simulink model "psb2rectifiers"  (Simulink 6.0)
settings: Solver=ode23tb  SolverMode=SingleTasking  StartTime=0.0  StopTime=0.1  RelTol=1e-3
InitFcn:
  | powericon('psbinitsys',bdroot);
libraries: powerlib2 x29
settings Model: Creator=sybille  LastModifiedBy=batserve  ExtModeTrigMode=oneshot  ExtModeArmWhenConnect=off  ExtModeAutoUpdateStatusClock=off
settings DataIOCC: LimitDataPoints=off  SignalLoggingName=sigsOut
settings OptimizationCC: BlockReduction=off  BooleanDataType=off
settings DebuggingCC: CheckExecutionContextPreStartOutputMsg=on  CheckExecutionContextRuntimeOutputMsg=on  SolverPrmCheckMsg=none
settings HardwareCC: TargetUnknown=on

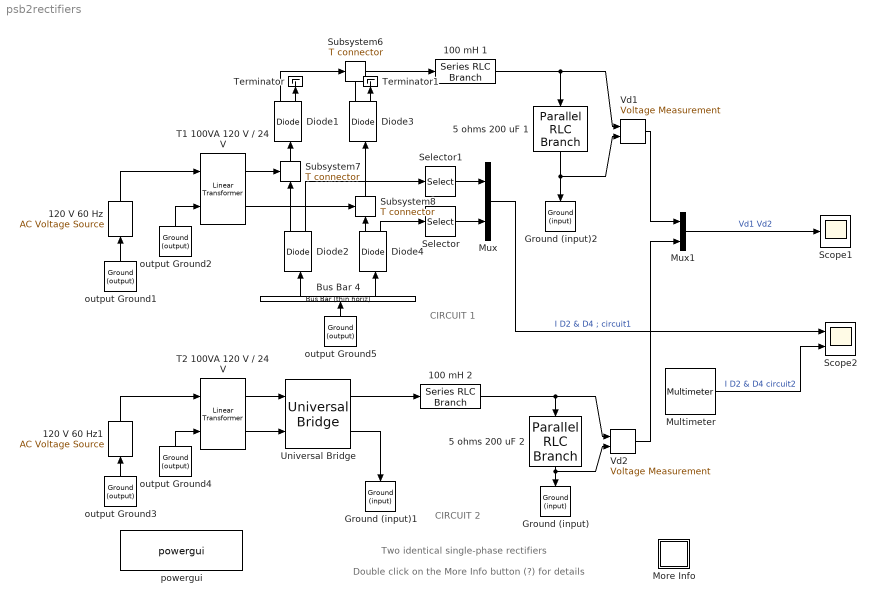
== system psb2rectifiers ==
  note: CIRCUIT 1
  note: Double click on the More Info button (?) for details
  note: CIRCUIT 2
  note: Two identical single-phase rectifiers
  100 mH 1 : powerlib2/Elements/Series RLC Branch  Tag=PoWeRsYsTeMbLoCk  a=0  b=100e-03  c=inf  mesure=None  PSBOutputType=1
  100 mH 2 : powerlib2/Elements/Series RLC Branch  Tag=PoWeRsYsTeMbLoCk  a=0  b=100e-03  c=inf  mesure=None  PSBOutputType=1
  120 V 60 Hz : powerlib2/Electrical Sources/AC Voltage Source  Tag=PoWeRsYsTeMbLoCk  Orientation=up  A=120*sqrt(2)  P=0  F=60  stime=0  mesure=None  PSBOutputType=1
  120 V 60 Hz1 : powerlib2/Electrical Sources/AC Voltage Source  Tag=PoWeRsYsTeMbLoCk  Orientation=up  A=120*sqrt(2)  P=0  F=60  stime=0  mesure=None  PSBOutputType=1
  5 ohms 200 uF 1 : powerlib2/Elements/Parallel RLC Branch  Tag=PoWeRsYsTeMbLoCk  Orientation=down  a=5  b=inf  c=200e-06  mesure=None  PSBOutputType=1
  5 ohms 200 uF 2 : powerlib2/Elements/Parallel RLC Branch  Tag=PoWeRsYsTeMbLoCk  Orientation=down  a=5  b=inf  c=200e-06  mesure=None  PSBOutputType=1
  Bus Bar 4 : powerlib2/Connectors/Bus Bar (thin horiz)  Tag=PoWeRsYsTeMbLoCk  Orientation=up  input=1  output=2  PSBOutputType=111111111111111111111111111111111111111111111111111111111111111111111111111111111111
  Diode{1..4} (4 alike) : powerlib2/Power Electronics/Diode  Tag=PoWeRsYsTeMbLoCk  Orientation=up  Ron=0.01  Lon=0  Vf=0.8  IC=0  Rs=250  Cs=0.1e-6  PSBOutputType=10
  Ground (input) : powerlib2/Connectors/Ground (input)  Tag=PoWeRsYsTeMbLoCk  Orientation=down
  Ground (input)1 : powerlib2/Connectors/Ground (input)  Tag=PoWeRsYsTeMbLoCk  Orientation=down
  Ground (input)2 : powerlib2/Connectors/Ground (input)  Tag=PoWeRsYsTeMbLoCk  Orientation=down
  More Info : Subsystem
      mask Display: disp('?')
  Multimeter : powerlib2/Measurements/Multimeter  Tag=PoWeRsYsTeMmEaSuReMeNt  PhasorSimulation=off  OutputType=Magnitude  sel=[2 4]  L=4  Gain=[1 1]  yselected={'Isw2: Universal Bridge','Isw4: Universal Bridge'};  PSBOutputType=1  PSBequivalent=0  AxesSetting=[0,0.1,-100,100]  Display=0  SavedBlockNames=-11
  Mux : Mux  Inputs=2
  Mux1 : Mux  Inputs=2
  Scope1 : Scope
      settings: TimeRange=0.1  YMin=0  YMax=20  SaveName=V2X  DataFormat=Array  SampleInput=on  SampleTime=10e-6
  Scope2 : Scope  NumInputPorts=2
      settings: TimeRange=0.1  YMin=0~0  YMax=4~4  SaveName=V2X  DataFormat=Array  SampleInput=on  SampleTime=10e-6
  Selector : Selector  InputPortWidth=2
  Selector1 : Selector  InputPortWidth=2
  Subsystem6 : powerlib2/Connectors/T connector  Tag=PoWeRsYsTeMbLoCk  PSBOutputType=1
  Subsystem7 : powerlib2/Connectors/T connector  Tag=PoWeRsYsTeMbLoCk  Orientation=up  PSBOutputType=1
  Subsystem8 : powerlib2/Connectors/T connector  Tag=PoWeRsYsTeMbLoCk  Orientation=up  PSBOutputType=1
  T1 100VA 120 V / 24 V : powerlib2/Elements/Linear Transformer  Tag=PoWeRsYsTeMbLoCk  a=[100 60]  b=[120 0.03 0.02]  c=[24 0.03 0.02]  w3check=off  d=[24 0.03 0.02]  e=[25 25]  mesure=None  PSBOutputType=1111
  T2 100VA 120 V / 24 V : powerlib2/Elements/Linear Transformer  Tag=PoWeRsYsTeMbLoCk  a=[100 60]  b=[120 0.03 0.02]  c=[24 0.03 0.02]  w3check=off  d=[24 0.03 0.02]  e=[25 25]  mesure=None  PSBOutputType=1111
  Terminator : Terminator
      settings: Orientation=up
  Terminator1 : Terminator
      settings: Orientation=up
  Universal Bridge : powerlib2/Power Electronics/Universal Bridge  Tag=PoWeRsYsTeMbLoCk  arms=2  confi=ABC as input terminals  injcc=250  cf=0.1e-6  device=Diodes  Ron=0.01  Lon=0  VFs="[  0.8  0.8  ]"  Vf=0.8  gtoparameters=[ 10e-6 , 20e-6 ]  igbtparameters=[ 1e-6 , 2e-6 ]  mesure=Device currents  PSBOutputType=111
  Vd1 : powerlib2/Measurements/Voltage Measurement  Tag=PoWeRsYsTeMmEaSuReMeNt  PhasorSimulation=off  OutputType=Magnitude  PSBOutputType=0  PSBequivalent=0
  Vd2 : powerlib2/Measurements/Voltage Measurement  Tag=PoWeRsYsTeMmEaSuReMeNt  PhasorSimulation=off  OutputType=Magnitude  PSBOutputType=0  PSBequivalent=0
  output Ground{1..5} (5 alike) : powerlib2/Connectors/Ground (output)  Tag=PoWeRsYsTeMbLoCk  Orientation=up  PSBOutputType=1
  powergui : powerlib2/powergui  Frange=[0:2:500]  Ylog=off  Xlog=on  save=off  variable=ZData  ZoomFFT=on  StartTime=0.0  cycles=1  DisplayStyle=off  fundamental=60  FreqAxis=off  MaxFrequency=1000  frequencyindice=1  frequencyindicesteady=1  RmsSteady=1  display=off  Ts=50e-6  methode=off  frequency=60  echomessages=off
  wires:
  Diode2/1 -> Subsystem7/1
  Bus Bar 4/1 -> Diode2/1
  120 V 60 Hz/1 -> T1 100VA 120 V / 24 V/1
  output Ground1/1 -> 120 V 60 Hz/1
  output Ground2/1 -> T1 100VA 120 V / 24 V/2
  Diode4/1 -> Subsystem8/1
  T1 100VA 120 V / 24 V/2 -> Subsystem8/Enable
  Bus Bar 4/2 -> Diode4/1
  Selector1/1 -> Mux/1
  Selector/1 -> Mux/2
  Diode4/2 -> Selector/1
  Diode2/2 -> Selector1/1
  T1 100VA 120 V / 24 V/1 -> Subsystem7/Enable
  Subsystem7/1 -> Diode1/1
  Diode3/1 -> Subsystem6/Enable
  Diode1/1 -> Subsystem6/1
  Subsystem6/1 -> 100 mH 1/1
  Subsystem8/1 -> Diode3/1
  120 V 60 Hz1/1 -> T2 100VA 120 V / 24 V/1
  output Ground3/1 -> 120 V 60 Hz1/1
  output Ground4/1 -> T2 100VA 120 V / 24 V/2
  T2 100VA 120 V / 24 V/2 -> Universal Bridge/2
  T2 100VA 120 V / 24 V/1 -> Universal Bridge/1
  Universal Bridge/2 -> Ground (input)1/1
  5 ohms 200 uF 2/1 -> Ground (input)/1, Vd2/2
  Universal Bridge/1 -> 100 mH 2/1
  100 mH 2/1 -> 5 ohms 200 uF 2/1, Vd2/1
  Mux/1 -> Scope2/1  "I D2 & D4 ; circuit1"
  Multimeter/1 -> Scope2/2  "I D2 & D4 circuit2"
  output Ground5/1 -> Bus Bar 4/1
  100 mH 1/1 -> 5 ohms 200 uF 1/1, Vd1/1
  5 ohms 200 uF 1/1 -> Vd1/2, Ground (input)2/1
  Mux1/1 -> Scope1/1  "Vd1 Vd2"
  Vd1/1 -> Mux1/1
  Vd2/1 -> Mux1/2
  Diode3/2 -> Terminator1/1
  Diode1/2 -> Terminator/1

== system psb2rectifiers/More Info ==
  note: This demonstration illustrates use of the Universal Bridge, Multimeter,
      | and Discrete System blocks
  note: Demonstration
  note: Circuit Description
  note: This system contains two identical circuits showing the operation of a single phase rectifier.
      |
      | The rectifiers are fed by a 120 V/ 24 V linear transformer. The rectified voltage is filtered by a
      | 100 mH / 200 uF filter and applied to a 5 ohm resistive load.
      | The load voltages are measured by two Voltage Measurement blocks Vd1 and Vd2.
      |
      | The top circuit (circuit 1) uses four individual diodes connected in a bridge configuration.
      | The currents of diodes 2 and 4 are obtained at the measurement 'm' output of the diode blocks
      | and sent to input 1 of Scope 2 through Selector and Multiplex blocks.
      |
      | The bottom circuit (circuit 2) is functiunally identical to circuit 1,
      | but the circuit assembly is considerably simplified by the use of the Universal Bridge.
  note: Open the Universal Bridge dialog box and notice that in order to obtain a four-diode bridge configuration,
      | the Power electronic devices field has been set to 'Diodes' and  that the number of arms has been set to 2.
      | Also, observe that the Measurements field has been set to 'Device currents', thus allowing
      | measurement of  diode currents through the Multimeter block.
      |
      | Now, double click on the Multimeter block. The four diode currents are listed in the left column.
      | Notice that only currents in diodes 2 and 4 have been selected and transferred in the right column.
      | The number of available signals at the multimeter output (2) is displayed on the block icon.
      |
      | Open the two scopes and start the simulation.
      | Compare the two load voltages Vd1 and Vd2 which are superimposed on Scope1.
      | Also, compare on Scope2 the currents flowing in diodes 2 and 4  for  circuit 1 and circuit 2.
      |
      | Notice that the circuit has been discretized by means of the Powergui  block.
      | The sample time (50e-6 s) appears on the block icon.
      |
      | Now, open the Powergui block and  deselect  "Discretize electrical model" .  The continuous ode23tb solver specified
      | in the Simulation parameters will now be used.  Restart the simulation and compare the continuous simulation results
      |  with the previous simulation results obtained with a discretized system.
  note: G. Sybille (Hydro-Quebec)
